simulink model "Integration_Forward_JFK_Line_Search"  (R2015a)
settings: Solver=ode3  StartTime=0.0  StopTime=500  FixedStep=0.01  MaxStep=0.01  RelTol=1e-3
values from neighbouring files (symbols this model uses):
  H0 = interp1q(Periodic_Solution(:,1),Periodic_Solution(:,4),time_shift(nn))    [Gradient_Descent_Spontaneous_Sleeping.m]
  I_update = I    [Gradient_Descent_Spontaneous_Sleeping.m]
  n0 = interp1q(Periodic_Solution(:,1),Periodic_Solution(:,7),time_shift(nn))    [Gradient_Descent_Spontaneous_Sleeping.m]
  Periodic_Solution = Periodic_Solution(Initial_Time*100+1:end,:)    [Gradient_Descent_Spontaneous_Sleeping.m]
  tol = 0.01    [Gradient_Descent_Spontaneous_Sleeping.m]
  x0 = interp1q(Periodic_Solution(:,1),Periodic_Solution(:,2),time_shift(nn))    [Gradient_Descent_Spontaneous_Sleeping.m]
  xc0 = interp1q(Periodic_Solution(:,1),Periodic_Solution(:,3),time_shift(nn))    [Gradient_Descent_Spontaneous_Sleeping.m]
settings Model: Creator=wangf7  LastModifiedBy=Jiawei Yin
settings OptimizationCC: ExpressionDepthLimit=2147483647
settings DebuggingCC: AlgebraicLoopMsg=none  ArtificialAlgebraicLoopMsg=none  UnderspecifiedInitializationDetection=Classic  MergeDetectMultiDrivingBlocksExec=none  SolverPrmCheckMsg=warning  StateNameClashWarn=warning

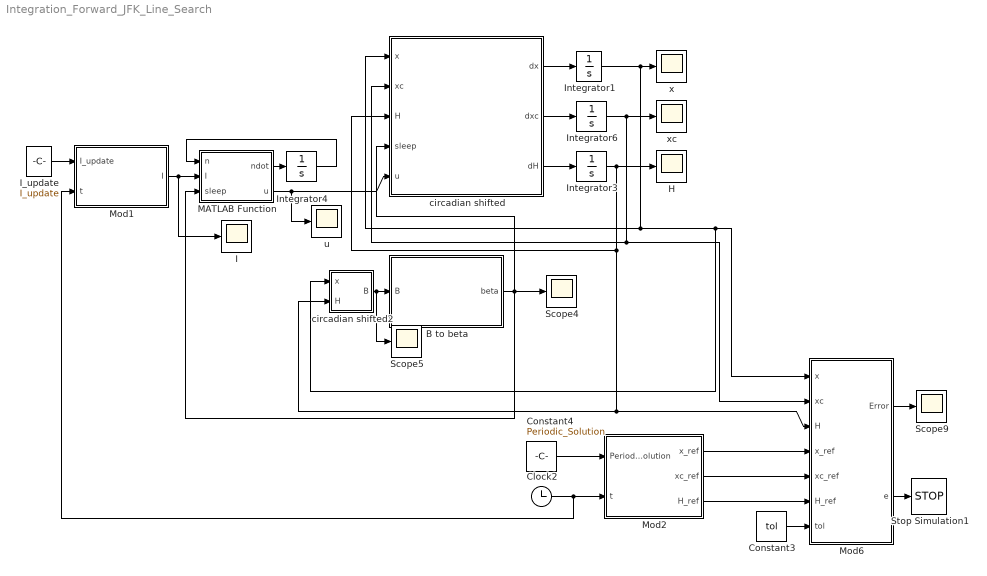
== system Integration_Forward_JFK_Line_Search ==
  "B to beta " : Subsystem
  Clock2 : Clock
  Constant3 : Constant  Value=tol
  Constant4 : Constant  Value=Periodic_Solution
  H : Scope
      settings: TimeRange=auto  MaxDataPoints=5000  SaveName=H_plus  YMin=0.00957  YMax=0.70084  SampleTime=-1  DataFormat=Array
  I : Scope
      settings: TimeRange=auto  MaxDataPoints=5000  SaveName=I_plus  YMin=-1250.00000  YMax=11250.00000  SampleTime=-1  DataFormat=Array
  I_update : Constant  Value=I_update
  Integrator1 : Integrator  InitialCondition=x0
  Integrator3 : Integrator  InitialCondition=H0
  Integrator4 : Integrator  InitialCondition=n0
  Integrator6 : Integrator  InitialCondition=xc0
  MATLAB Function : MATLAB Function  TreatAsAtomicUnit=on
      settings: PermitHierarchicalResolution=ParametersOnly
  Mod1 : MATLAB Function  TreatAsAtomicUnit=on
      settings: PermitHierarchicalResolution=ParametersOnly
  Mod2 : MATLAB Function  TreatAsAtomicUnit=on
      settings: PermitHierarchicalResolution=ParametersOnly
  Mod6 : MATLAB Function  TreatAsAtomicUnit=on
      settings: PermitHierarchicalResolution=ParametersOnly
  Scope4 : Scope
      settings: TimeRange=auto  MaxDataPoints=5000  SaveName=sleep_plus  YMin=-1.00000  YMax=1.00000  SampleTime=-1  DataFormat=Array
  Scope5 : Scope
      settings: TimeRange=auto  MaxDataPoints=5000  SaveName=B_plus  YMin=0.09109  YMax=0.29109  SampleTime=-1  DataFormat=Array
  Scope9 : Scope
      settings: TimeRange=auto  MaxDataPoints=5000  SaveName=Error_plus  YMin=0.06228  YMax=0.08228  SampleTime=-1  DataFormat=Array
  Stop Simulation1 : Stop
  circadian shifted : MATLAB Function  TreatAsAtomicUnit=on
      settings: PermitHierarchicalResolution=ParametersOnly
  circadian shifted2 : MATLAB Function  TreatAsAtomicUnit=on
      settings: PermitHierarchicalResolution=ParametersOnly
  u : Scope
      settings: TimeRange=auto  MaxDataPoints=5000  SaveName=u_plus  YMin=-0.21608  YMax=1.94475  SampleTime=-1  DataFormat=Array
  x : Scope
      settings: TimeRange=auto  MaxDataPoints=5000  SaveName=x_plus  YMin=-0.81237  YMax=-0.61237  SampleTime=-1  DataFormat=Array
  xc : Scope
      settings: TimeRange=auto  MaxDataPoints=5000  SaveName=xc_plus  YMin=0.62881  YMax=0.82881  SampleTime=-1  DataFormat=Array
  wires:
  circadian shifted/1(dx) -> Integrator1/1
  Integrator1/1 -> x/1, circadian shifted2/1(x), Mod6/1(x), circadian shifted/1(x)
  Integrator6/1 -> Mod6/2(xc), circadian shifted/2(xc), xc/1
  circadian shifted2/1(B) -> Scope5/1, "B to beta "/1(B)
  "B to beta "/1(beta) -> MATLAB Function/3(sleep), Scope4/1, circadian shifted/4(sleep)
  Constant4/1 -> Mod2/1(Periodic_Solution)
  Clock2/1 -> Mod1/2(t), Mod2/2(t)
  Mod6/2(e) -> Stop Simulation1/1
  Mod6/1(Error) -> Scope9/1
  Mod2/3(H_ref) -> Mod6/6(H_ref)
  Constant3/1 -> Mod6/7(tol)
  circadian shifted/2(dxc) -> Integrator6/1
  circadian shifted/3(dH) -> Integrator3/1
  Integrator3/1 -> circadian shifted2/2(H), Mod6/3(H), circadian shifted/3(H), H/1
  Mod2/1(x_ref) -> Mod6/4(x_ref)
  Mod2/2(xc_ref) -> Mod6/5(xc_ref)
  MATLAB Function/2(u) -> u/1, circadian shifted/5(u)
  I_update/1 -> Mod1/1(I_update)
  MATLAB Function/1(ndot) -> Integrator4/1
  Integrator4/1 -> MATLAB Function/1(n)
  Mod1/1(I) -> I/1, MATLAB Function/2(I)

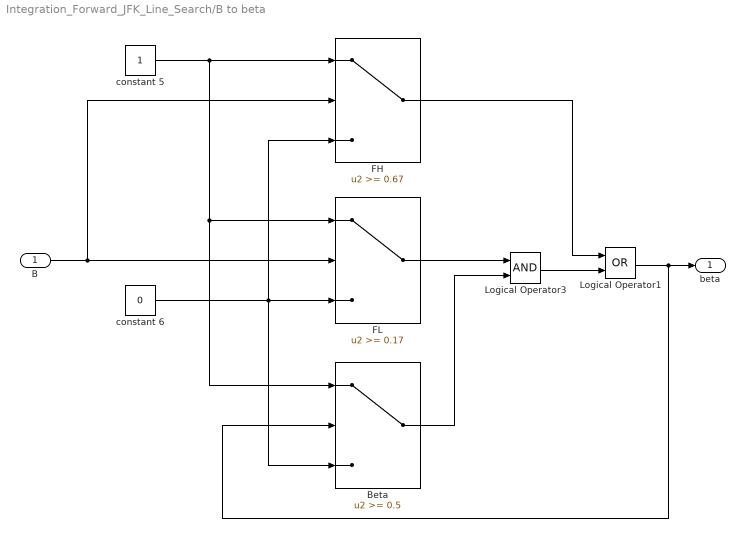
== system Integration_Forward_JFK_Line_Search/B to beta  ==
  B : Inport
  Beta : Switch  Threshold=0.5
  FH : Switch  Threshold=0.67
  FL : Switch  Threshold=0.17
  Logical Operator1 : Logic  Operator=OR  AllPortsSameDT=off  OutDataTypeStr=boolean
  Logical Operator3 : Logic  AllPortsSameDT=off  OutDataTypeStr=boolean
  constant 5 : Constant
  constant 6 : Constant  Value=0
  beta : Outport
  wires:
  constant 5/1 -> Beta/1, FL/1, FH/1
  constant 6/1 -> Beta/3, FH/3, FL/3
  B/1 -> FH/2, FL/2
  Logical Operator1/1 -> Beta/2, beta/1
  FL/1 -> Logical Operator3/1
  Beta/1 -> Logical Operator3/2
  Logical Operator3/1 -> Logical Operator1/2
  FH/1 -> Logical Operator1/1

== matlab function Integration_Forward_JFK_Line_Search/Mod1 ==
  data: I_update input; I output; t input
function I  = fcn(I_update,t)
%#codegen
if t<I_update(end,1)
    I=interp1q(I_update(:,1),I_update(:,2),t);
else
    I=I_update(end,2);
end

== matlab function Integration_Forward_JFK_Line_Search/MATLAB Function ==
  data: n input; I input; ndot output; u output; sleep input
function [ndot,u] = fcn(n,I,sleep)
G=33.75;
alpha0=0.05;
beta=0.0075;
I0=9500;

alpha=alpha0*(I/I0)^0.5;
u=G*alpha*(1-n)*(1-sleep);
ndot=60*[alpha*(1-n)*(1-sleep)-beta*n];

== matlab function Integration_Forward_JFK_Line_Search/circadian shifted ==
  data: x input; xc input; H input; sleep input; u input; dx output; dxc output; dH output
function [ dx,dxc,dH] = fcn(x,xc,H,sleep,u)
%#eml

tr=18.2;
td=4.2;

q = 1/3;
taux = 24.2;
k = 0.55;
mu=0.13;

B = u*(1-sleep)*(1-0.4*x)*(1-0.4*xc)*(1-sleep);

dx = (pi/12)*(xc + B  + mu*(1/3*x + 4/3*x^3 - 256/105*x^7));
dxc = (pi/12)*(q*B *xc - (24/(taux*0.99729))^2*x - k*B*x);
dH = (1-sleep)*(1-H)/tr-(H*sleep)/td;

== matlab function Integration_Forward_JFK_Line_Search/circadian shifted2 ==
  data: x input; H input; B output
function B = fcn(x,H)
%#eml
B=H-0.1333*x;

== matlab function Integration_Forward_JFK_Line_Search/Mod2 ==
  data: Periodic_Solution input; x_ref output; xc_ref output; t input; H_ref output
function [x_ref,xc_ref,H_ref] = fcn(Periodic_Solution,t)
%#codegen
x_ref=interp1q(Periodic_Solution(:,1),Periodic_Solution(:,2),t);
xc_ref=interp1q(Periodic_Solution(:,1),Periodic_Solution(:,3),t);
H_ref=interp1q(Periodic_Solution(:,1),Periodic_Solution(:,4),t);
% sleep_ref=interp1q(Periodic_Solution(:,1),Periodic_Solution(:,6),t);

== matlab function Integration_Forward_JFK_Line_Search/Mod6 ==
  data: Error output; x input; xc input; H input; x_ref input; xc_ref input; e output; H_ref input; tol input
function [Error,e] = fcn(x,xc,H,x_ref,xc_ref,H_ref,tol)
%#codegen
Error=(H-H_ref)^2+(x-x_ref)^2+(xc-xc_ref)^2;
e=Error<tol;
